simulink model "VE_EPRM_24_25"  (R2022b)
settings: Solver=ode4  StartTime=0  StopTime=200  FixedStep=1e-4  RelTol=1e-3  EnableMultiTasking=on
values from neighbouring files (symbols this model uses):
  CYCL =     [cycle_ECE.mat]
undefined symbols (not defined in the file or in its folder): cel_serie, cx, f, g, ke, ki, Kie, Kpe, Kpm, kred, Lmcc, mod_serie, Mv, n, nconv, r, Rcell, rho, Rmcc, S, Voc, Vv
libraries: slpidlib x1, simulink x1
settings Model: Creator=Tony  LastModifiedBy=ZinouAb
settings SolverCC: AlgebraicLoopSolver=TrustRegion
settings DataIOCC: SaveFormat=Array  SignalLoggingSaveFormat=ModelDataLogs  ReturnWorkspaceOutputs=off  SignalLoggingName=sigsOut
settings OptimizationCC: BooleanDataType=off  ExpressionDepthLimit=2147483647  LifeSpan=inf
settings DebuggingCC: SaveWithParameterizedLinksMsg=none  UnderspecifiedInitializationDetection=Classic  MergeDetectMultiDrivingBlocksExec=none  SignalResolutionControl=TryResolveAllWithWarning  MultiTaskDSMMsg=warning  MultiTaskCondExecSysMsg=none  FcnCallInpInsideContextMsg=warning  UnconnectedInputMsg=warning  UnconnectedOutputMsg=warning  UnconnectedLineMsg=warning  StateNameClashWarn=warning  SFUnexpectedBacktrackingDiag=warning  SFNoUnconditionalDefaultTransitionDiag=warning  SFExecutionAtInitializationDiag=none  SFMachineParentedDataDiag=warning  ArithmeticOperatorsInVariantConditions=warning
settings HardwareCC: ProdBitPerPointer=32  ProdBitPerSizeT=32  ProdBitPerPtrDiffT=32  ProdLargestAtomicFloat=None  ProdIntDivRoundTo=Undefined  ProdEndianess=Unspecified  ProdWordSize=32  ProdHWDeviceType=32-bit Generic  TargetUnknown=on
settings ModelReferenceCC: EnableRefExpFcnMdlSchedulingChecks=on  PropagateSignalLabelsOutOfModel=off
settings SFSimCC: SimUseLocalCustomCode=off  CustomCodeUndefinedFunction=UseInterfaceOnly
settings RTWCC: RTWUseLocalCustomCode=off
settings CodeAppCC: StateflowObjectComments=on
settings GRTTargetCC: TargetLangStandard=C89/C90 (ANSI)  CombineOutputUpdateFcns=off  GRTInterface=on
settings ConfigComp: CovMetricSettings=dw  CovSaveCumulativeToWorkspaceVar=on  CovSaveSingleToWorkspaceVar=on

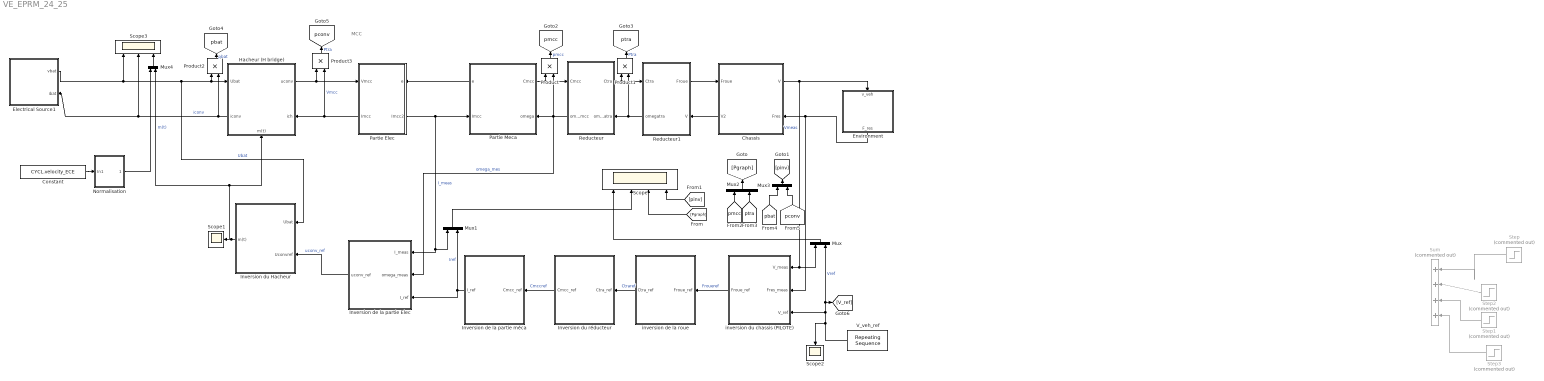
== system VE_EPRM_24_25 ==
  note: MCC
  Chassis : Subsystem
      settings: PortSchema="{\"entries\":[{\"content\":{\"sides\":[{\"content\":{\"connectorIds\":[\"In1\",\"Out2\"]},\"type\":\"ConnectorPlacement.EquallySpacedRectSide\",\"uuid\":\"2a4fefbc-7af2-45ac-94e1-720f9d1a181b\"},{\"content\":{\"connectorIds\":[\"Out1\",\"In2\"],\"side\":\"RIGHT\"},\"type\":\"ConnectorPlacement.EquallySpacedRectSide\",\"uuid\":\"47213f8a-38f1-43b2-8885-5842ee71090a\"},{\"content\":{\"connectorIds\":[],\"side\":\"TOP\"},\"type\":\"ConnectorPlacement.EquallySpacedRectSide\",\"uuid\":\"9ff55915-a798-409c-870e-d15a860382f9\"}]},\"type\":\"ConnectorPlacement.EquallySpacedConnector\",\"uuid\":\"647a32d4-94be-4190-bdc8-90a1a32d4cbf\"}],\"packageUris\":[\"http://schema.mathworks.com/mf0/Connector/R2020b\"],\"version\":\"1.0\"}"
      mask Display: plot(0,0,100,100,[10,10,90,90,10],[90,10,10,90,90], [10,90],[10,90])
  Constant : Constant  Value=CYCL.velocity_ECE
  Electrical Source1 : Subsystem
      settings: PortSchema="{\"entries\":[{\"content\":{\"sides\":[{\"content\":{\"connectorIds\":[]},\"type\":\"ConnectorPlacement.EquallySpacedRectSide\",\"uuid\":\"0447c061-d881-4364-8bf9-5f237b3f85a5\"},{\"content\":{\"connectorIds\":[\"Out1\",\"In1\"],\"side\":\"RIGHT\"},\"type\":\"ConnectorPlacement.EquallySpacedRectSide\",\"uuid\":\"63637e17-0c1c-4ae6-b384-822c77d172cb\"},{\"content\":{\"connectorIds\":[],\"side\":\"TOP\"},\"type\":\"ConnectorPlacement.EquallySpacedRectSide\",\"uuid\":\"c198568a-ae39-4bd1-be2e-5ec17640e827\"}]},\"type\":\"ConnectorPlacement.EquallySpacedConnector\",\"uuid\":\"4bbe213b-1f87-4d3e-871e-0040a2c9184f\"}],\"packageUris\":[\"http://schema.mathworks.com/mf0/Connector/R2020b\"],\"version\":\"1.0\"}"
      mask Display:
      | plot(0,0,100,100, 1.2*[50,57.68,60.77,63.08,64.97,66.58,68,69.26,70.4, 	71.42,72.36,78.28,80,78.28,72.36,71.42,70.4, 	69.26,68,66.58,64.97,63.08,60.77,57.68,50,42.32, 	39.23,36.92,35.03,33.42,32,30.74,29.6,28.58, 	27.64,21.72,20,21.72,27.64,28.58,29.6,30.74,32, 	33.42,35.03,36.92,39.23,42.32,50]-10, 1.2*[20,21,22,23,24,25,26,27,28,29,30,40,50,60,70,71,72, 	73,74,75,76,77,78,79,80,79,78,77,76,75,74,73,72, 	71,70,60,50,40,30,29,28,27,26,25,24,23,22,21,20]-10)
      | disp('ES')
  Environment : Subsystem  AncestorBlock=simulink/REM/SE
      settings: LibrarySourceBlock=simulink/REM/SE
      mask Display:
      | plot(0,0,100,100, 1.2*[50,57.68,60.77,63.08,64.97,66.58,68,69.26,70.4, 	71.42,72.36,78.28,80,78.28,72.36,71.42,70.4, 	69.26,68,66.58,64.97,63.08,60.77,57.68,50,42.32, 	39.23,36.92,35.03,33.42,32,30.74,29.6,28.58, 	27.64,21.72,20,21.72,27.64,28.58,29.6,30.74,32, 	33.42,35.03,36.92,39.23,42.32,50]-10, 1.2*[20,21,22,23,24,25,26,27,28,29,30,40,50,60,70,71,72, 	73,74,75,76,77,78,79,80,79,78,77,76,75,74,73,72, 	71,70,60,50,40,30,29,28,27,26,25,24,23,22,21,20]-10)
      | disp('ROAD')
  Hacheur (H bridge) : Subsystem
      settings: PortSchema="{\"entries\":[{\"content\":{\"sides\":[{\"content\":{\"connectorIds\":[\"In1\",\"Out2\"]},\"type\":\"ConnectorPlacement.EquallySpacedRectSide\",\"uuid\":\"15c37a82-4fae-4dd0-ab5a-78fb718c05e2\"},{\"content\":{\"connectorIds\":[\"Out1\",\"In3\"],\"side\":\"RIGHT\"},\"type\":\"ConnectorPlacement.EquallySpacedRectSide\",\"uuid\":\"2898708c-5198-4fba-9c94-abd5bb9e9c70\"},{\"content\":{\"connectorIds\":[],\"side\":\"TOP\"},\"type\":\"ConnectorPlacement.EquallySpacedRectSide\",\"uuid\":\"a769b592-c34b-45c3-8b04-17631095b399\"},{\"content\":{\"connectorIds\":[\"In2\"],\"side\":\"BOTTOM\"},\"type\":\"ConnectorPlacement.EquallySpacedRectSide\",\"uuid\":\"3f87bc4b-31a4-497c-9119-c9de1168f7cf\"}]},\"type\":\"ConnectorPlacement.EquallySpacedConnector\",\"uuid\":\"cf4da0bd-1e1f-410f-93a1-c54772eba95e\"}],\"packageUris\":[\"http://schema.mathworks.com/mf0/Connector/R2020b\"],\"version\":\"1.0\"}"
      mask Display: plot(0,0,100,100,[10,10,90,90,10],[90,10,10,90,90])
  Inversion de la partie Elec : Subsystem  AncestorBlock=simulink/SMC/Asservissement Correcteur IP
      settings: LibrarySourceBlock=|
      | simulink/SMC/Asservissement
      | Correcteur IP
      mask Display: plot(0,0,100,100, [10,30,90,70,10,90],[90,10,10,90,90,10])
  Inversion de la partie méca : Subsystem  AncestorBlock=simulink/SMC/Inversion EC avec mesure
      settings: LibrarySourceBlock=|
      | simulink/SMC/Inversion EC
      | avec mesure
      mask Display: plot(0,0,100,100,[10,30,90,70,10],[90,10,10,90,90])
  Inversion du Hacheur : Subsystem  AncestorBlock=simulink/SMC/Inversion EC avec mesure
      settings: LibrarySourceBlock=|
      | simulink/SMC/Inversion EC
      | avec mesure
      mask Display: plot(0,0,100,100,[10,30,90,70,10],[90,10,10,90,90])
  Inversion du réducteur : Subsystem  AncestorBlock=simulink/SMC/Inversion EC avec mesure
      settings: LibrarySourceBlock=|
      | simulink/SMC/Inversion EC
      | avec mesure
      mask Display: plot(0,0,100,100,[10,30,90,70,10],[90,10,10,90,90])
  Mux{,1..4} (5 alike) : Mux  Inputs=2
  Normalisation : Subsystem
  Partie Elec : Subsystem
      settings: PortSchema="{\"entries\":[{\"content\":{\"sides\":[{\"content\":{\"connectorIds\":[\"In1\",\"Out2\"]},\"type\":\"ConnectorPlacement.EquallySpacedRectSide\",\"uuid\":\"2a4fefbc-7af2-45ac-94e1-720f9d1a181b\"},{\"content\":{\"connectorIds\":[\"In2\",\"Out1\"],\"side\":\"RIGHT\"},\"type\":\"ConnectorPlacement.EquallySpacedRectSide\",\"uuid\":\"47213f8a-38f1-43b2-8885-5842ee71090a\"},{\"content\":{\"connectorIds\":[],\"side\":\"TOP\"},\"type\":\"ConnectorPlacement.EquallySpacedRectSide\",\"uuid\":\"9ff55915-a798-409c-870e-d15a860382f9\"}]},\"type\":\"ConnectorPlacement.EquallySpacedConnector\",\"uuid\":\"647a32d4-94be-4190-bdc8-90a1a32d4cbf\"}],\"packageUris\":[\"http://schema.mathworks.com/mf0/Connector/R2020b\"],\"version\":\"1.0\"}"
      mask Display: plot(0,0,100,100,[10,10,90,90,10],[90,10,10,90,90], [10,90],[10,90])
  Partie Meca : Subsystem
      settings: PortSchema="{\"entries\":[{\"content\":{\"sides\":[{\"content\":{\"connectorIds\":[\"Out2\",\"In1\"]},\"type\":\"ConnectorPlacement.EquallySpacedRectSide\",\"uuid\":\"2a4fefbc-7af2-45ac-94e1-720f9d1a181b\"},{\"content\":{\"connectorIds\":[\"Out1\",\"In2\"],\"side\":\"RIGHT\"},\"type\":\"ConnectorPlacement.EquallySpacedRectSide\",\"uuid\":\"47213f8a-38f1-43b2-8885-5842ee71090a\"},{\"content\":{\"connectorIds\":[],\"side\":\"TOP\"},\"type\":\"ConnectorPlacement.EquallySpacedRectSide\",\"uuid\":\"9ff55915-a798-409c-870e-d15a860382f9\"}]},\"type\":\"ConnectorPlacement.EquallySpacedConnector\",\"uuid\":\"647a32d4-94be-4190-bdc8-90a1a32d4cbf\"}],\"packageUris\":[\"http://schema.mathworks.com/mf0/Connector/R2020b\"],\"version\":\"1.0\"}"
      mask Display: plot(0,0,100,100, 1.4*[50,57.68,60.77,63.08,64.97,66.58,68,69.26,70.4, 	71.42,72.36,78.28,80,78.28,72.36,71.42,70.4, 	69.26,68,66.58,64.97,63.08,60.77,57.68,50,42.32, 	39.23,36.92,35.03,33.42,32,30.74,29.6,28.58, 	27.64,21.72,20,21.72,27.64,28.58,29.6,30.74,32, 	33.42,35.03,36.92,39.23,42.32,50]-20, 1.4*[20,21,22,23,24,25,26,27,28,29,30,40,50,60,70,71,72, 	73,74,75,76,77,78,79,80,79,78,77,76,75,74,73,72, 	71,70,60,50,40,30,29,28,27,26,25,24,23,22,21,20]-20)
  Product{,1..3} (4 alike) : Product
  Reducteur : Subsystem
      settings: PortSchema="{\"entries\":[{\"content\":{\"sides\":[{\"content\":{\"connectorIds\":[\"In1\",\"Out2\"]},\"type\":\"ConnectorPlacement.EquallySpacedRectSide\",\"uuid\":\"e4ebbfb6-8d69-4e28-b674-770b062d5c59\"},{\"content\":{\"connectorIds\":[\"Out1\",\"In2\"],\"side\":\"RIGHT\"},\"type\":\"ConnectorPlacement.EquallySpacedRectSide\",\"uuid\":\"824a92d3-cd27-40c6-b343-dc2eefca7831\"},{\"content\":{\"connectorIds\":[],\"side\":\"TOP\"},\"type\":\"ConnectorPlacement.EquallySpacedRectSide\",\"uuid\":\"a5f3f993-294a-4e41-8967-8e26580e0c28\"}]},\"type\":\"ConnectorPlacement.EquallySpacedConnector\",\"uuid\":\"a532f145-12bc-495c-8c35-d0598d698f25\"}],\"packageUris\":[\"http://schema.mathworks.com/mf0/Connector/R2020b\"],\"version\":\"1.0\"}"
      mask Display: plot(0,0,100,100,[10,10,90,90,10],[90,10,10,90,90])
  Reducteur1 : Subsystem
      settings: PortSchema="{\"entries\":[{\"content\":{\"sides\":[{\"content\":{\"connectorIds\":[\"In1\",\"Out2\"]},\"type\":\"ConnectorPlacement.EquallySpacedRectSide\",\"uuid\":\"e4ebbfb6-8d69-4e28-b674-770b062d5c59\"},{\"content\":{\"connectorIds\":[\"Out1\",\"In2\"],\"side\":\"RIGHT\"},\"type\":\"ConnectorPlacement.EquallySpacedRectSide\",\"uuid\":\"824a92d3-cd27-40c6-b343-dc2eefca7831\"},{\"content\":{\"connectorIds\":[],\"side\":\"TOP\"},\"type\":\"ConnectorPlacement.EquallySpacedRectSide\",\"uuid\":\"a5f3f993-294a-4e41-8967-8e26580e0c28\"}]},\"type\":\"ConnectorPlacement.EquallySpacedConnector\",\"uuid\":\"a532f145-12bc-495c-8c35-d0598d698f25\"}],\"packageUris\":[\"http://schema.mathworks.com/mf0/Connector/R2020b\"],\"version\":\"1.0\"}"
      mask Display: plot(0,0,100,100,[10,10,90,90,10],[90,10,10,90,90])
  Scope : Scope  NumInputPorts=4
  Scope1 : Scope
  Scope2 : Scope
  Scope3 : Scope  NumInputPorts=3
  Step : Step  Commented=on  Time=10  After=10  SampleTime=0
  Step1 : Step  Commented=on  Time=30  SampleTime=0
  Step2 : Step  Commented=on  Time=20  After=-20  SampleTime=0
  Step3 : Step  Commented=on  Time=40  After=-40  SampleTime=0
  Sum : Sum  Commented=on  Inputs=|++++
  V_veh_ref : simulink/Sources/Repeating Sequence  rep_seq_t=CYCL.time_ECE  rep_seq_y=CYCL.velocity_ECE
  inversion de la roue : Subsystem  AncestorBlock=simulink/SMC/Inversion EC avec mesure
      settings: LibrarySourceBlock=|
      | simulink/SMC/Inversion EC
      | avec mesure
      mask Display: plot(0,0,100,100,[10,30,90,70,10],[90,10,10,90,90])
  inversion du chassis (PILOTE) : Subsystem  AncestorBlock=simulink/SMC/Asservissement Correcteur IP
      settings: LibrarySourceBlock=|
      | simulink/SMC/Asservissement
      | Correcteur IP
      mask Display: plot(0,0,100,100, [10,30,90,70,10,90],[90,10,10,90,90,10])
  tag scope: pbat=global, pconv=global, pmcc=global, ptra=global
  wires:
  Partie Meca/2(e) -> Partie Elec/2(e)
  Chassis/2(V2) -> Reducteur1/2(V)
  Chassis/1(V) -> Mux/1, inversion du chassis (PILOTE)/1(V_meas), Environment/1(v_veh)  "Vmeas"
  Environment/1(F_res) -> inversion du chassis (PILOTE)/2(Fres_meas), Chassis/2(Fres)
  Inversion du Hacheur/1(m(t)) -> Mux4/2, Hacheur (H bridge)/2(m(t)), Scope1/1  "m(t)"
  Partie Elec/1(Imcc2) -> Mux1/1, Inversion de la partie Elec/1(I_meas), Partie Meca/1(Imcc)  "I_meas"
  Partie Meca/1(Cmcc) -> Reducteur/1(Cmcc), Product/1
  Reducteur/1(Ctra) -> Reducteur1/1(Ctra), Product1/1
  Reducteur1/2(omegatra) -> Reducteur/2(omegatra), Product1/2
  Reducteur1/1(Froue) -> Chassis/1(Froue)
  Reducteur/2(omegamcc) -> Inversion de la partie Elec/2(omega_meas), Partie Meca/2(omega), Product/2  "omega_mes"
  V_veh_ref/1 -> Scope2/1, inversion du chassis (PILOTE)/3(V_ref), Mux/2, [V_ref]  "Vref"
  inversion du chassis (PILOTE)/1(Froue_ref) -> inversion de la roue/1(Froue_ref)  "Froueref"
  inversion de la roue/1(Ctra_ref) -> Inversion du réducteur/1(Ctra_ref)  "Ctraref"
  Inversion du réducteur/1(Cmcc_ref) -> Inversion de la partie méca/1(Cmcc_ref)  "Cmccref"
  Inversion de la partie Elec/1(uconv_ref) -> Inversion du Hacheur/2("Uconvref ")  "uconv_ref"
  Mux/1 -> Scope/1
  Inversion de la partie méca/1(I_ref) -> Inversion de la partie Elec/3(I_ref), Mux1/2  "Iref"
  Partie Elec/2(Imcc) -> Hacheur (H bridge)/3("ich "), Product3/2  "Vmcc"
  Mux1/1 -> Scope/2
  Mux2/1 -> [Pgraph]
  [Pgraph] -> Scope/3
  Step1/1 -> Sum/3
  Step3/1 -> Sum/4
  Step2/1 -> Sum/2
  Step/1 -> Sum/1
  Product2/1 -> [pbat]  "pbat"
  Hacheur (H bridge)/2(iconv) -> Scope3/2, Electrical Source1/1(ibat), Product2/2  "iconv"
  Mux3/1 -> [pinv]
  Electrical Source1/1(vbat) -> Inversion du Hacheur/1(Ubat), Hacheur (H bridge)/1("Ubat "), Product2/1, Scope3/1  "Ubat"
  Hacheur (H bridge)/1("uconv ") -> Partie Elec/1(Vmcc), Product3/1
  [pinv] -> Scope/4
  Product/1 -> [pmcc]  "pmcc"
  Product1/1 -> [ptra]  "Ptra"
  [pmcc] -> Mux2/1
  [ptra] -> Mux2/2
  Product3/1 -> [pconv]  "Ptra"
  [pbat] -> Mux3/1
  [pconv] -> Mux3/2
  Mux4/1 -> Scope3/3
  Constant/1 -> Normalisation/1(In1)
  Normalisation/1(V_norm) -> Mux4/1

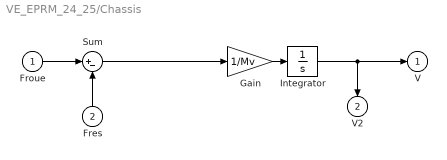
== system VE_EPRM_24_25/Chassis ==
  Froue : Inport
  Fres : Inport  Port=2
  Gain : Gain  Gain=1/Mv
  Integrator : Integrator
  Sum : Sum  Inputs=|+-
  V : Outport  InitialOutput=0
  V2 : Outport  Port=2  InitialOutput=0
  wires:
  Integrator/1 -> V2/1, V/1
  Froue/1 -> Sum/1
  Gain/1 -> Integrator/1
  Fres/1 -> Sum/2
  Sum/1 -> Gain/1

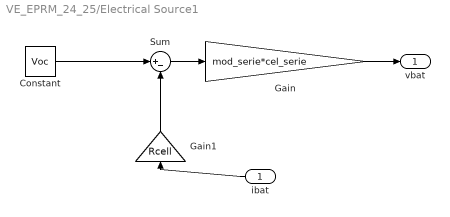
== system VE_EPRM_24_25/Electrical Source1 ==
  ibat : Inport
  Constant : Constant  Value=Voc
  Gain : Gain  Gain=mod_serie*cel_serie
  Gain1 : Gain  Gain=Rcell
  Sum : Sum  Inputs=|+-
  vbat : Outport
  wires:
  Constant/1 -> Sum/1
  Sum/1 -> Gain/1
  ibat/1 -> Gain1/1
  Gain/1 -> vbat/1
  Gain1/1 -> Sum/2

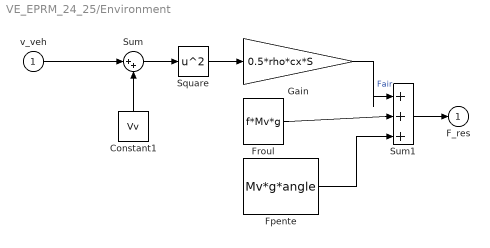
== system VE_EPRM_24_25/Environment ==
  v_veh : Inport
  Constant1 : Constant  Value=Vv
  Fpente : Constant  Value=Mv*g*angle
  Froul : Constant  Value=f*Mv*g
  Gain : Gain  Gain=0.5*rho*cx*S
  Square : Math  Operator=square  SignedPower=on
  Sum : Sum  Inputs=|++
  Sum1 : Sum  Inputs=|+++
  F_res : Outport  InitialOutput=0
  wires:
  v_veh/1 -> Sum/1
  Constant1/1 -> Sum/2
  Sum/1 -> Square/1
  Square/1 -> Gain/1
  Gain/1 -> Sum1/1  "Fair"
  Froul/1 -> Sum1/2
  Fpente/1 -> Sum1/3
  Sum1/1 -> F_res/1

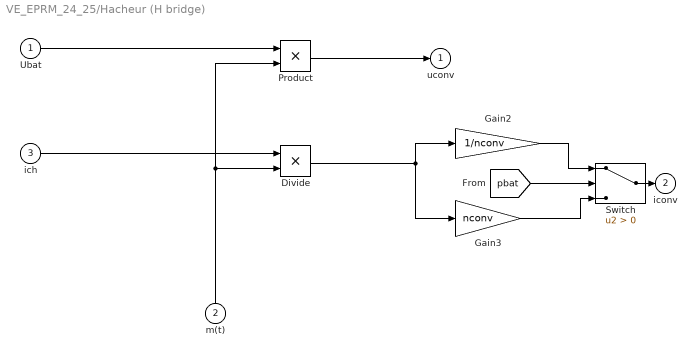
== system VE_EPRM_24_25/Hacheur (H bridge) ==
  "Ubat " : Inport
  m(t) : Inport  Port=2
  "ich " : Inport  Port=3
  Divide : Product  Inputs=**
  Gain2 : Gain  Gain=1/nconv
  Gain3 : Gain  Gain=nconv
  Product : Product
  Switch : Switch  Criteria=u2 > Threshold  SaturateOnIntegerOverflow=off  InputSameDT=off
  "uconv " : Outport  InitialOutput=0
  iconv : Outport  Port=2  InitialOutput=0
  wires:
  m(t)/1 -> Divide/2, Product/2
  "Ubat "/1 -> Product/1
  "ich "/1 -> Divide/1
  Product/1 -> "uconv "/1
  [pbat] -> Switch/2
  Gain2/1 -> Switch/1
  Divide/1 -> Gain3/1, Gain2/1
  Gain3/1 -> Switch/3
  Switch/1 -> iconv/1

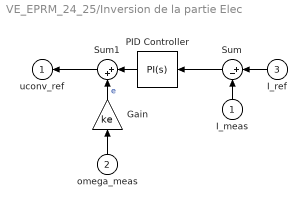
== system VE_EPRM_24_25/Inversion de la partie Elec ==
  I_meas : Inport
  omega_meas : Inport  Port=2
  I_ref : Inport  Port=3
  Gain : Gain  Gain=ke
  PID Controller : slpidlib/PID Controller  Controller=PI  Form=Parallel  TimeDomain=Continuous-time  UseExternalTs=off  SampleTime=-1  IntegratorMethod=Forward Euler  FilterMethod=Forward Euler  ControllerParametersSource=internal  P=Kpe  I=Kie  UseKiTs=off  D=0  N=100  UseFilter=on  TunerSelectOption=Transfer Function Based (PID Tuner App)  InitialConditionSource=internal  InitialConditionForIntegrator=0  InitialConditionForFilter=0  DifferentiatorICPrevScaledInput=0  ExternalReset=none  TrackingMode=off  Kt=1  LimitOutput=off  SatLimitsSource=internal  UpperSaturationLimit=inf  LowerSaturationLimit=-inf  LinearizeAsGain=on  AntiWindupMode=none  Kb=1  LimitIntegrator=off  UpperIntegratorSaturationLimit=inf  LowerIntegratorSaturationLimit=-inf  POutMin=[]  POutMax=[]  IOutMin=[]  IOutMax=[]  DOutMin=[]  DOutMax=[]  NOutMin=[]  NOutMax=[]  SumOutMin=[]  SumOutMax=[]  SaturationOutMin=[]  SaturationOutMax=[]  PParamMin=[]  PParamMax=[]  IParamMin=[]  IParamMax=[]  DParamMin=[]  DParamMax=[]  NParamMin=[]  NParamMax=[]  KbParamMin=[]  KbParamMax=[]  KtParamMin=[]  KtParamMax=[]  KbOutMin=[]  KbOutMax=[]  KtOutMin=[]  KtOutMax=[]  IntegratorOutMin=[]  IntegratorOutMax=[]  FilterOutMin=[]  FilterOutMax=[]  SumI1OutMin=[]  SumI1OutMax=[]  SumI2OutMin=[]  SumI2OutMax=[]  SumI3OutMin=[]  SumI3OutMax=[]  SumI4OutMin=[]  SumI4OutMax=[]  SumDOutMin=[]  SumDOutMax=[]  DifferentiatorOutMin=[]  DifferentiatorOutMax=[]  FilterDiffOutCoefMin=[]  FilterDiffOutCoefMax=[]  ReciprocalOutMin=[]  ReciprocalOutMax=[]  SumDenOutMin=[]  SumDenOutMax=[]  SumNumOutMin=[]  SumNumOutMax=[]  DivideOutMin=[]  DivideOutMax=[]  UdiffTsProdOutMin=[]  UdiffTsProdOutMax=[]  NTsProdOutMin=[]  NTsProdOutMax=[]  UintegralTsProdOutMin=[]  UintegralTsProdOutMax=[]  UngainTsProdOutMin=[]  UngainTsProdOutMax=[]  ClampingZeroOutDataTypeStr=Inherit: Inherit via back propagation  ClampingZeroOutMin=[]  ClampingZeroOutMax=[]  FilterDenConstantOutDataTypeStr=Inherit: Inherit via back propagation  FilterDenConstantOutMin=[]  FilterDenConstantOutMax=[]  PCopyOutDataTypeStr=Inherit: Inherit via back propagation  PCopyOutMin=[]  PCopyOutMax=[]  NCopyOutDataTypeStr=Inherit: Inherit via back propagation  NCopyOutMin=[]  NCopyOutMax=[]  IntegratorContinuousStateAttributes=''  IntegratorStateMustResolveToSignalObject=off  IntegratorRTWStateStorageClass=Auto  FilterContinuousStateAttributes=''  FilterStateMustResolveToSignalObject=off  FilterRTWStateStorageClass=Auto  ParallelPVariant=InternalParameters  IdealPVariant=Disabled  IVariant=InternalParameters  DVariant=Disabled  IntegratorVariant=Continuous  SatVariant=Disabled  AWVariant=Passthrough  PCopyVariant=Disabled  TRVariant=Disabled  FdbkBlocksVariant=Forward  IdealPFdbkVariant=Disabled  SatFdbkVariant=Disabled  DerivativeFilterVariant=Disabled  NVariant=Disabled  NCopyVariant=Disabled_SignalSpec  FilterICVariant=Disabled  IntegratorICVariant=InternalICs  ExternalResetVariant=Disabled  TRSumVariant=Passthrough  SumFdbkVariant=Disabled  SumVariant=Sum_PI  TsampFilterVariant=InternalTs  TsampNgainVariant=Passthrough  TsampIntegralVariant=Passthrough  ExternalSaturationOutDataTypeStr=Inherit: Same as second input
  Sum : Sum  Inputs=|+-
  Sum1 : Sum  Inputs=|++
  uconv_ref : Outport  InitialOutput=0
  wires:
  I_meas/1 -> Sum/2
  omega_meas/1 -> Gain/1
  Sum/1 -> PID Controller/1
  Sum1/1 -> uconv_ref/1
  Gain/1 -> Sum1/2  "e"
  PID Controller/1 -> Sum1/1
  I_ref/1 -> Sum/1

== system VE_EPRM_24_25/Inversion de la partie méca ==
  Cmcc_ref : Inport
  Gain : Gain  Gain=1/ki
  I_ref : Outport  InitialOutput=0
  wires:
  Cmcc_ref/1 -> Gain/1
  Gain/1 -> I_ref/1

== system VE_EPRM_24_25/Inversion du Hacheur ==
  Ubat : Inport
  "Uconvref " : Inport  Port=2
  Divide : Product  Inputs=*/
  Memory : Memory  InitialCondition=48
  m(t) : Outport  InitialOutput=0
  wires:
  Ubat/1 -> Memory/1
  Divide/1 -> m(t)/1
  "Uconvref "/1 -> Divide/1
  Memory/1 -> Divide/2

== system VE_EPRM_24_25/Inversion du réducteur ==
  Ctra_ref : Inport
  Gain : Gain  Gain=1/kred
  Cmcc_ref : Outport  InitialOutput=0
  wires:
  Gain/1 -> Cmcc_ref/1
  Ctra_ref/1 -> Gain/1

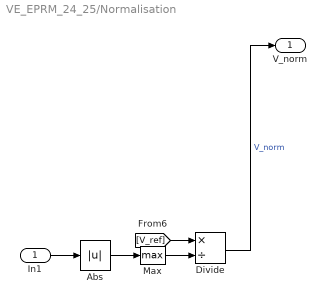
== system VE_EPRM_24_25/Normalisation ==
  In1 : Inport
  Abs : Abs  SaturateOnIntegerOverflow=off
  Divide : Product  Inputs=*/
  Max : MinMax  Function=max
  V_norm : Outport
  wires:
  Divide/1 -> V_norm/1  "V_norm"
  Abs/1 -> Max/1
  Max/1 -> Divide/2
  [V_ref] -> Divide/1
  In1/1 -> Abs/1

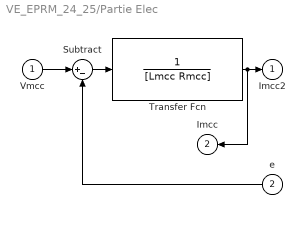
== system VE_EPRM_24_25/Partie Elec ==
  Vmcc : Inport
  e : Inport  Port=2
  Subtract : Sum  Inputs=|+-
  Transfer Fcn : TransferFcn  Denominator=[Lmcc Rmcc]
  Imcc2 : Outport  InitialOutput=0
  Imcc : Outport  Port=2  InitialOutput=0
  wires:
  Transfer Fcn/1 -> Imcc/1, Imcc2/1
  e/1 -> Subtract/2
  Subtract/1 -> Transfer Fcn/1
  Vmcc/1 -> Subtract/1

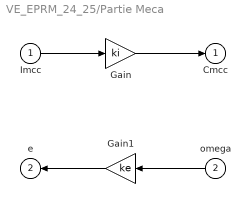
== system VE_EPRM_24_25/Partie Meca ==
  Imcc : Inport
  omega : Inport  Port=2
  Gain : Gain  Gain=ki
  Gain1 : Gain  Gain=ke
  Cmcc : Outport  InitialOutput=0
  e : Outport  Port=2  InitialOutput=0
  wires:
  omega/1 -> Gain1/1
  Imcc/1 -> Gain/1
  Gain1/1 -> e/1
  Gain/1 -> Cmcc/1

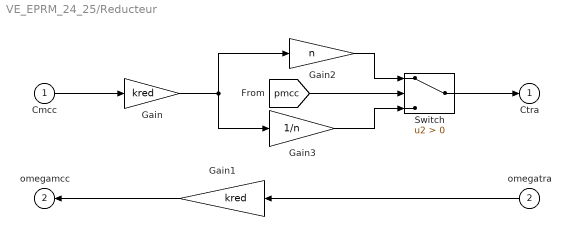
== system VE_EPRM_24_25/Reducteur ==
  Cmcc : Inport
  omegatra : Inport  Port=2
  Gain : Gain  Gain=kred
  Gain1 : Gain  Gain=kred
  Gain2 : Gain  Gain=n
  Gain3 : Gain  Gain=1/n
  Switch : Switch  Criteria=u2 > Threshold  SaturateOnIntegerOverflow=off  InputSameDT=off
  Ctra : Outport  InitialOutput=0
  omegamcc : Outport  Port=2  InitialOutput=0
  wires:
  Gain/1 -> Gain3/1, Gain2/1
  Switch/1 -> Ctra/1
  omegatra/1 -> Gain1/1
  Gain2/1 -> Switch/1
  [pmcc] -> Switch/2
  Cmcc/1 -> Gain/1
  Gain3/1 -> Switch/3
  Gain1/1 -> omegamcc/1

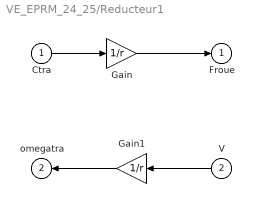
== system VE_EPRM_24_25/Reducteur1 ==
  Ctra : Inport
  V : Inport  Port=2
  Gain : Gain  Gain=1/r
  Gain1 : Gain  Gain=1/r
  Froue : Outport  InitialOutput=0
  omegatra : Outport  Port=2  InitialOutput=0
  wires:
  Gain/1 -> Froue/1
  V/1 -> Gain1/1
  Ctra/1 -> Gain/1
  Gain1/1 -> omegatra/1

== system VE_EPRM_24_25/inversion de la roue ==
  Froue_ref : Inport
  Gain : Gain  Gain=r
  Ctra_ref : Outport  InitialOutput=0
  wires:
  Froue_ref/1 -> Gain/1
  Gain/1 -> Ctra_ref/1

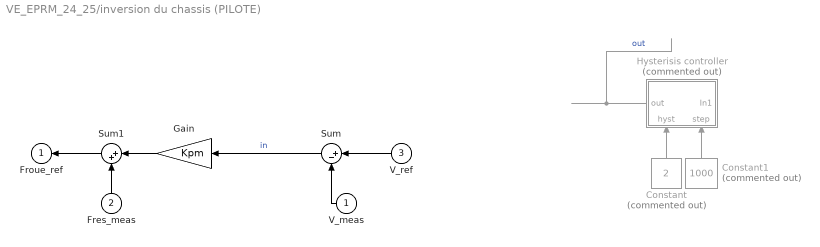
== system VE_EPRM_24_25/inversion du chassis (PILOTE) ==
  V_meas : Inport
  Fres_meas : Inport  Port=2
  V_ref : Inport  Port=3
  Constant : Constant  Commented=on  Value=2
  Constant1 : Constant  Commented=on  Value=1000
  Gain : Gain  Gain=Kpm
  Hysterisis controller : Subsystem  Commented=on
      settings: PortSchema="{\"entries\":[{\"content\":{\"sides\":[{\"content\":{\"connectorIds\":[\"In1\"]},\"type\":\"ConnectorPlacement.EquallySpacedRectSide\",\"uuid\":\"f66aa083-2ee8-4426-b441-0f8ce3c91bc6\"},{\"content\":{\"connectorIds\":[\"Out1\"],\"side\":\"RIGHT\"},\"type\":\"ConnectorPlacement.EquallySpacedRectSide\",\"uuid\":\"e535ff9d-11f2-429a-8d26-bff265e6dce4\"},{\"content\":{\"connectorIds\":[\"In2\",\"In3\"],\"side\":\"TOP\"},\"type\":\"ConnectorPlacement.EquallySpacedRectSide\",\"uuid\":\"3bf3f486-5ffc-4655-8aef-50265858aab1\"},{\"content\":{\"connectorIds\":[],\"side\":\"BOTTOM\"},\"type\":\"ConnectorPlacement.EquallySpacedRectSide\",\"uuid\":\"619b2421-7bbc-4c41-b693-a17d0c478cc9\"}]},\"type\":\"ConnectorPlacement.EquallySpacedConnector\",\"uuid\":\"4c23f3cf-154a-4c58-b671-46cc18db332d\"}],\"packageUris\":[\"http://schema.mathworks.com/mf0/Connector/R2020b\"],\"version\":\"1.0\"}"
  Sum : Sum  Inputs=|+-
  Sum1 : Sum  Inputs=|++
  Froue_ref : Outport  InitialOutput=0
  wires:
  Hysterisis controller/1(out) -> ?  "out"
  Sum/1 -> Gain/1  "in"
  Constant/1 -> Hysterisis controller/3(hyst)
  Fres_meas/1 -> Sum1/2
  Sum1/1 -> Froue_ref/1
  ? -> Hysterisis controller/1(In1)  "in"
  Constant1/1 -> Hysterisis controller/2(step)
  V_ref/1 -> Sum/1
  V_meas/1 -> Sum/2
  Gain/1 -> Sum1/1

== system VE_EPRM_24_25/inversion du chassis (PILOTE)/Hysterisis controller ==
  In1 : Inport
  step : Inport  Port=2
  hyst : Inport  Port=3
  MATLAB Function : MATLAB Function  TreatAsAtomicUnit=on
  Memory : Memory
  out : Outport
  wires:
  In1/1 -> Memory/1, MATLAB Function/1(u)  "input"
  Memory/1 -> MATLAB Function/2(uprev)
  MATLAB Function/1(out) -> out/1
  step/1 -> MATLAB Function/4(step)
  hyst/1 -> MATLAB Function/3(hyst)

== matlab function VE_EPRM_24_25/inversion du chassis (PILOTE)/Hysterisis controller/MATLAB Function ==
  data: u input; out output; uprev input; hyst input; step input
function out = hystcontrol(u,uprev,hyst,step)

if u>hyst
    out= uprev-step;
elseif u<hyst
    out= uprev+step;
else
    out=uprev;

end
